simulink model "parte3_ex1"  (R2021b)
settings: Solver=VariableStepAuto  StartTime=0.0  StopTime=6  RelTol=1e-3
values from neighbouring files (symbols this model uses):
  h = 0.03    [parte3_script.m]
  Jm = 1.3475e-6    (= 1.3475e-06)    [parte3_script.m]
  Ke = 0.0159    [parte3_script.m]
  Kf = 0.000001176    (= 1.176e-06)    [parte3_script.m]
  L = Laa(2:end)    [parte3_script.m]
  La = 0    [parte3_script.m]
  Lc = L1/(1-polo_i)    [parte3_script.m]
  Ra = 8    [parte3_script.m]
undefined symbols (not defined in the file or in its folder): DiscIntNeverNeededParam
settings Model: Creator=Dylan  LastModifiedBy=Dylan

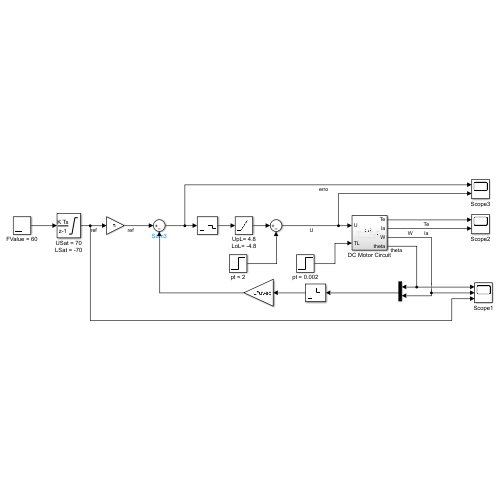
[thumbnail: Simulink's stored preview of the top-level diagram]
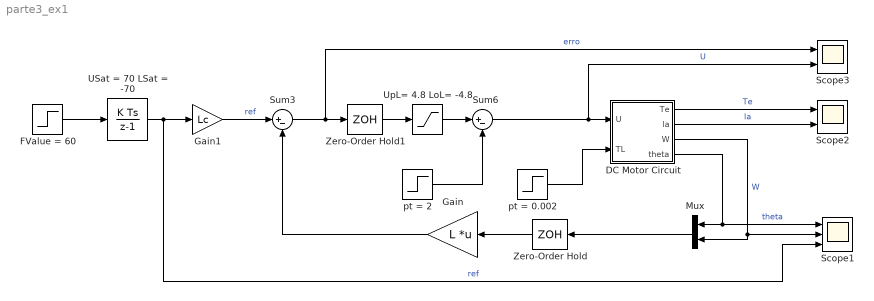
== system parte3_ex1 ==
  DC Motor Circuit : Subsystem
  FValue = 60 : Step  After=60  SampleTime=0
  Gain : Gain  Gain=L  Multiplication=Matrix(K*u) (u vector)
  Gain1 : Gain  Gain=Lc
  Mux : Mux  Inputs=2
  Scope1 : Scope  NumInputPorts=3
  Scope2 : Scope  NumInputPorts=2
  Scope3 : Scope  NumInputPorts=2
  Sum3 : Sum  Inputs=|+-
  Sum6 : Sum  Inputs=|+-
  USat = 70 LSat = -70 : DiscreteIntegrator  SampleTime=h  LimitOutput=on  UpperSaturationLimit=70  LowerSaturationLimit=-70  ICPrevOutput=DiscIntNeverNeededParam  ICPrevScaledInput=DiscIntNeverNeededParam
  UpL= 4.8 LoL= -4.8 : Saturate  UpperLimit=4.8  LowerLimit=-4.8
  Zero-Order Hold : ZeroOrderHold  SampleTime=h
  Zero-Order Hold1 : ZeroOrderHold  SampleTime=h
  pt = 0.002 : Step  Time=4  After=0.002  SampleTime=0
  pt = 2 : Step  Time=5  After=2  SampleTime=0
  wires:
  pt = 0.002/1 -> DC Motor Circuit/2(TL)
  Sum3/1 -> Scope3/1, Zero-Order Hold1/1  "erro"
  FValue = 60/1 -> USat = 70 LSat = -70/1
  USat = 70 LSat = -70/1 -> Scope1/3, Gain1/1  "ref"
  Zero-Order Hold/1 -> Gain/1
  Sum6/1 -> Scope3/2, DC Motor Circuit/1(U)  "U"
  DC Motor Circuit/3(W) -> Mux/2, Scope1/2  "W"
  Mux/1 -> Zero-Order Hold/1
  Gain/1 -> Sum3/2
  pt = 2/1 -> Sum6/2
  Gain1/1 -> Sum3/1  "ref"
  DC Motor Circuit/1(Te) -> Scope2/1  "Te"
  DC Motor Circuit/2(la) -> Scope2/2  "la"
  DC Motor Circuit/4(theta) -> Mux/1, Scope1/1  "theta"
  UpL= 4.8 LoL= -4.8/1 -> Sum6/1
  Zero-Order Hold1/1 -> UpL= 4.8 LoL= -4.8/1

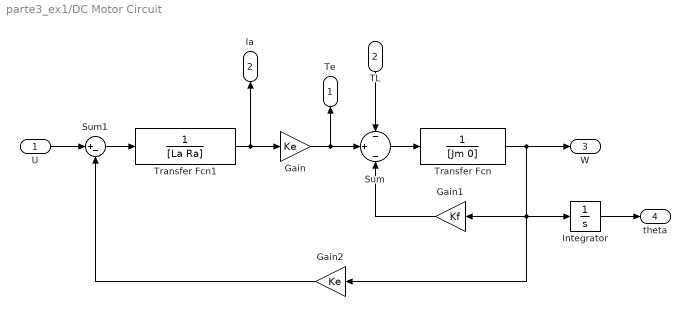
== system parte3_ex1/DC Motor Circuit ==
  U : Inport
  TL : Inport  Port=2
  Gain : Gain  Gain=Ke
  Gain1 : Gain  Gain=Kf
  Gain2 : Gain  Gain=Ke
  Integrator : Integrator
  Sum : Sum  Inputs=-|+|-
  Sum1 : Sum  Inputs=|+-
  Transfer Fcn : TransferFcn  Denominator=[Jm 0]
  Transfer Fcn1 : TransferFcn  Denominator=[La Ra]
  Te : Outport
  la : Outport  Port=2
  W : Outport  Port=3
  theta : Outport  Port=4
  wires:
  U/1 -> Sum1/1
  Transfer Fcn/1 -> W/1, Gain2/1, Integrator/1, Gain1/1
  Transfer Fcn1/1 -> la/1, Gain/1
  Gain2/1 -> Sum1/2
  Sum/1 -> Transfer Fcn/1
  Gain/1 -> Te/1, Sum/2
  TL/1 -> Sum/1
  Gain1/1 -> Sum/3
  Sum1/1 -> Transfer Fcn1/1
  Integrator/1 -> theta/1
